simulink model "sim_pmsm"  (R2024b)
settings: Solver=VariableStepAuto  StartTime=0.0  StopTime=10.0  RelTol=1e-3
settings Model: Creator=27abd  LastModifiedBy=27abd

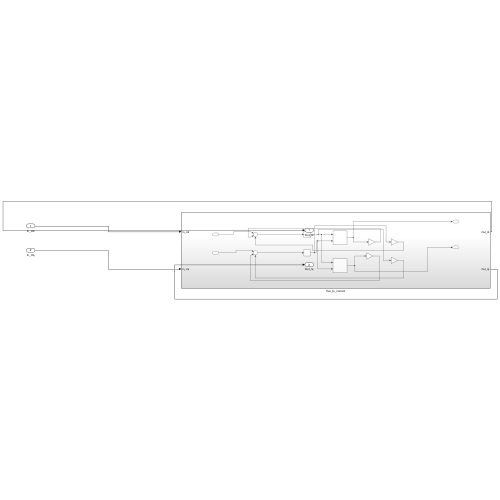
[thumbnail: Simulink's stored preview of the top-level diagram]
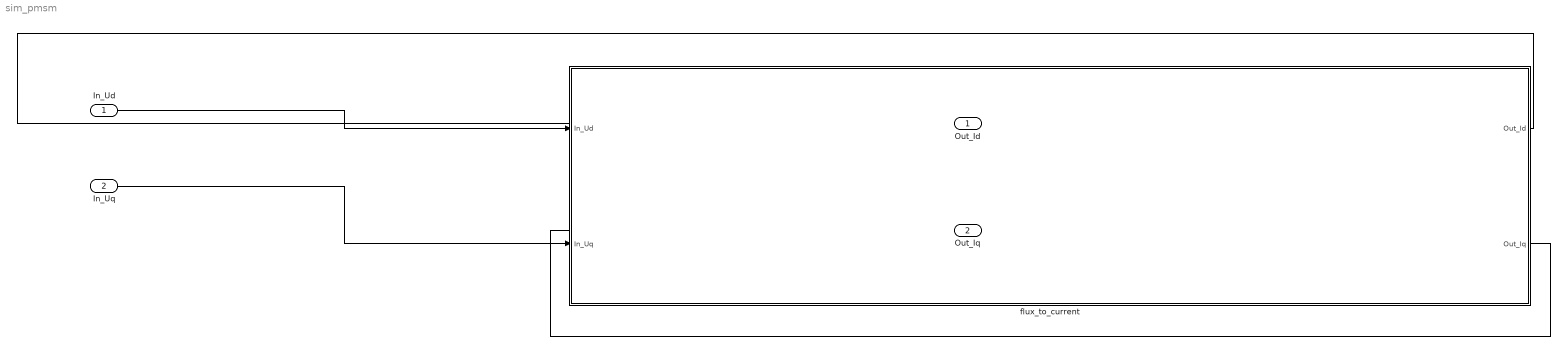
== system sim_pmsm ==
  In_Ud : Inport
  In_Uq : Inport  Port=2
  flux_to_current : Subsystem
  Out_Id : Outport
  Out_Iq : Outport  Port=2
  wires:
  In_Ud/1 -> flux_to_current/1(In_Ud)
  In_Uq/1 -> flux_to_current/2(In_Uq)
  flux_to_current/1(Out_Id) -> Out_Id/1
  flux_to_current/2(Out_Iq) -> Out_Iq/1

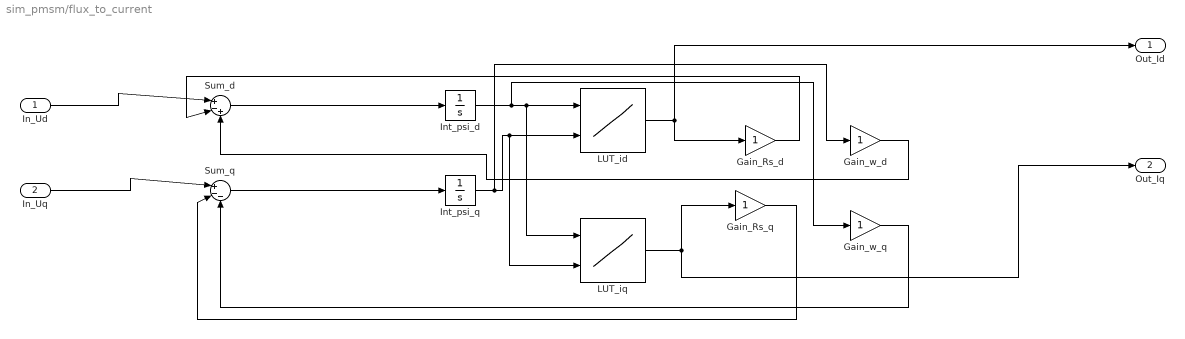
== system sim_pmsm/flux_to_current ==
  In_Ud : Inport
  In_Uq : Inport  Port=2
  Gain_Rs_d : Gain
  Gain_Rs_q : Gain
  Gain_w_d : Gain
  Gain_w_q : Gain
  Int_psi_d : Integrator
  Int_psi_q : Integrator
  LUT_id : Lookup_n-D  BreakpointsForDimension1=[1:3]  BreakpointsForDimension2=[1:3]  InternalRulePriority=Speed  RndMeth=Simplest
      settings: InputPortMap=u0,u1
  LUT_iq : Lookup_n-D  BreakpointsForDimension1=[1:3]  BreakpointsForDimension2=[1:3]  InternalRulePriority=Speed  RndMeth=Simplest
      settings: InputPortMap=u0,u1
  Sum_d : Sum  Inputs=|+-+
  Sum_q : Sum  Inputs=|+--
  Out_Id : Outport
  Out_Iq : Outport  Port=2
  wires:
  Int_psi_q/1 -> Gain_w_d/1, LUT_iq/2, LUT_id/2
  Int_psi_d/1 -> Gain_w_q/1, LUT_iq/1, LUT_id/1
  Sum_q/1 -> Int_psi_q/1
  Gain_Rs_q/1 -> Sum_q/2
  LUT_iq/1 -> Out_Iq/1, Gain_Rs_q/1
  Sum_d/1 -> Int_psi_d/1
  In_Uq/1 -> Sum_q/1
  Gain_w_q/1 -> Sum_q/3
  Gain_Rs_d/1 -> Sum_d/2
  Gain_w_d/1 -> Sum_d/3
  In_Ud/1 -> Sum_d/1
  LUT_id/1 -> Out_Id/1, Gain_Rs_d/1
